simulink model "A4_1"  (R2022b)
settings: Solver=VariableStepAuto  StartTime=0.0  StopTime=10.0  RelTol=1e-3
values from neighbouring files (symbols this model uses):
  D = sqrt(D)/(2*pi)    [CD_head_modal_a3.m]    (also in PIDcode.m = T_d)
  I = 0.1    [Assignment_6.m]    (also in PIDcode.m = 1/T_i)
  N = 1/T_t    [PIDcode.m]
  P = Kp/3    [PIDcode.m]
undefined symbols (not defined in the file or in its folder): Xa1, Xa2, Xa3, Xa4, Zs1, Zs2, Zs3, Zs4
libraries: cstblocks x4, slpidlib x1
settings Model: Creator=Akshat  LastModifiedBy=aront

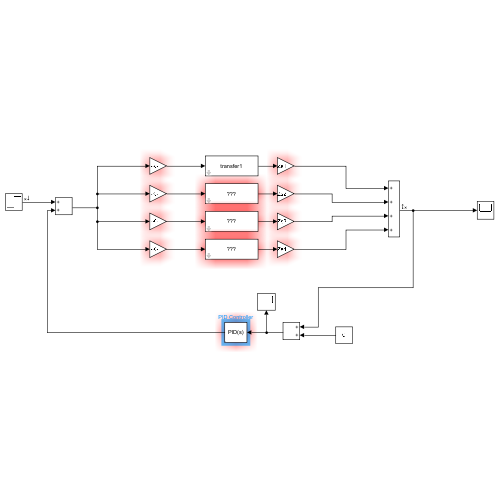
[thumbnail: Simulink's stored preview of the top-level diagram]
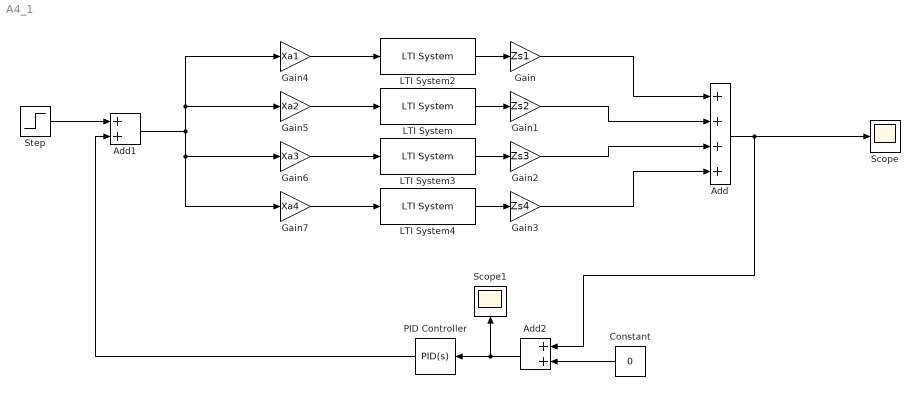
== system A4_1 ==
  Add : Sum  Inputs=++++
  Add1 : Sum
  Add2 : Sum
  Constant : Constant  Value=0
  Gain : Gain  Gain=Zs1
  Gain1 : Gain  Gain=Zs2
  Gain2 : Gain  Gain=Zs3
  Gain3 : Gain  Gain=Zs4
  Gain4 : Gain  Gain=Xa1
  Gain5 : Gain  Gain=Xa2
  Gain6 : Gain  Gain=Xa3
  Gain7 : Gain  Gain=Xa4
  LTI System : cstblocks/LTI System  sys=transfer2  IC=[]
  LTI System2 : cstblocks/LTI System  sys=transfer1  IC=[]
  LTI System3 : cstblocks/LTI System  sys=transfer3  IC=[]
  LTI System4 : cstblocks/LTI System  sys=transfer4  IC=[]
  PID Controller : slpidlib/PID Controller  Controller=PID  Form=Parallel  TimeDomain=Continuous-time  UseExternalTs=off  SampleTime=-1  IntegratorMethod=Forward Euler  FilterMethod=Forward Euler  ControllerParametersSource=internal  P=P  I=I  UseKiTs=off  D=D  N=N  UseFilter=on  TunerSelectOption=Transfer Function Based (PID Tuner App)  InitialConditionSource=internal  InitialConditionForIntegrator=0  InitialConditionForFilter=0  DifferentiatorICPrevScaledInput=0  ExternalReset=none  TrackingMode=off  Kt=1  LimitOutput=off  SatLimitsSource=internal  UpperSaturationLimit=inf  LowerSaturationLimit=-inf  LinearizeAsGain=on  AntiWindupMode=none  Kb=1  LimitIntegrator=off  UpperIntegratorSaturationLimit=inf  LowerIntegratorSaturationLimit=-inf  POutMin=[]  POutMax=[]  IOutMin=[]  IOutMax=[]  DOutMin=[]  DOutMax=[]  NOutMin=[]  NOutMax=[]  SumOutMin=[]  SumOutMax=[]  SaturationOutMin=[]  SaturationOutMax=[]  PParamMin=[]  PParamMax=[]  IParamMin=[]  IParamMax=[]  DParamMin=[]  DParamMax=[]  NParamMin=[]  NParamMax=[]  KbParamMin=[]  KbParamMax=[]  KtParamMin=[]  KtParamMax=[]  KbOutMin=[]  KbOutMax=[]  KtOutMin=[]  KtOutMax=[]  IntegratorOutMin=[]  IntegratorOutMax=[]  FilterOutMin=[]  FilterOutMax=[]  SumI1OutMin=[]  SumI1OutMax=[]  SumI2OutMin=[]  SumI2OutMax=[]  SumI3OutMin=[]  SumI3OutMax=[]  SumI4OutMin=[]  SumI4OutMax=[]  SumDOutMin=[]  SumDOutMax=[]  DifferentiatorOutMin=[]  DifferentiatorOutMax=[]  FilterDiffOutCoefMin=[]  FilterDiffOutCoefMax=[]  ReciprocalOutMin=[]  ReciprocalOutMax=[]  SumDenOutMin=[]  SumDenOutMax=[]  SumNumOutMin=[]  SumNumOutMax=[]  DivideOutMin=[]  DivideOutMax=[]  UdiffTsProdOutMin=[]  UdiffTsProdOutMax=[]  NTsProdOutMin=[]  NTsProdOutMax=[]  UintegralTsProdOutMin=[]  UintegralTsProdOutMax=[]  UngainTsProdOutMin=[]  UngainTsProdOutMax=[]  ClampingZeroOutDataTypeStr=Inherit: Inherit via back propagation  ClampingZeroOutMin=[]  ClampingZeroOutMax=[]  FilterDenConstantOutDataTypeStr=Inherit: Inherit via back propagation  FilterDenConstantOutMin=[]  FilterDenConstantOutMax=[]  PCopyOutDataTypeStr=Inherit: Inherit via back propagation  PCopyOutMin=[]  PCopyOutMax=[]  NCopyOutDataTypeStr=Inherit: Inherit via back propagation  NCopyOutMin=[]  NCopyOutMax=[]  IntegratorContinuousStateAttributes=''  IntegratorStateMustResolveToSignalObject=off  IntegratorRTWStateStorageClass=Auto  FilterContinuousStateAttributes=''  FilterStateMustResolveToSignalObject=off  FilterRTWStateStorageClass=Auto  ParallelPVariant=InternalParameters  IdealPVariant=Disabled  IVariant=InternalParameters  DVariant=InternalParameters  IntegratorVariant=Continuous  SatVariant=Disabled  AWVariant=Passthrough  PCopyVariant=Disabled  TRVariant=Disabled  FdbkBlocksVariant=Forward  IdealPFdbkVariant=Disabled  SatFdbkVariant=Disabled  DerivativeFilterVariant=ContFilter  NVariant=InternalParameters  NCopyVariant=Disabled  FilterICVariant=InternalICsFilter  IntegratorICVariant=InternalICs  ExternalResetVariant=Disabled  TRSumVariant=Passthrough  SumFdbkVariant=Disabled  SumVariant=Sum_PID  TsampFilterVariant=InternalTs  TsampNgainVariant=Passthrough  TsampIntegralVariant=Passthrough  ExternalSaturationOutDataTypeStr=Inherit: Same as second input
  Scope : Scope
  Scope1 : Scope
  Step : Step  Time=0.1  SampleTime=0
  wires:
  LTI System2/1 -> Gain/1
  LTI System/1 -> Gain1/1
  LTI System3/1 -> Gain2/1
  LTI System4/1 -> Gain3/1
  Gain/1 -> Add/1
  Gain1/1 -> Add/2
  Gain2/1 -> Add/3
  Gain3/1 -> Add/4
  Add1/1 -> Gain7/1, Gain6/1, Gain5/1, Gain4/1
  Gain4/1 -> LTI System2/1
  Gain5/1 -> LTI System/1
  Gain7/1 -> LTI System4/1
  Gain6/1 -> LTI System3/1
  Step/1 -> Add1/1
  PID Controller/1 -> Add1/2
  Add2/1 -> PID Controller/1, Scope1/1
  Add/1 -> Add2/1, Scope/1
  Constant/1 -> Add2/2
